simulink subsystem "StudentTemplate_NGCMAN017_M1"  (R2025a)
settings: Solver=VariableStepAuto  StartTime=0.0  StopTime=10.0  RelTol=1e-3
libraries: eeGeneralControl x3, simulink x2, slpidlib x1
settings Model: Creator=JesseJabezArendse  LastModifiedBy=Manelisi Ngcobo

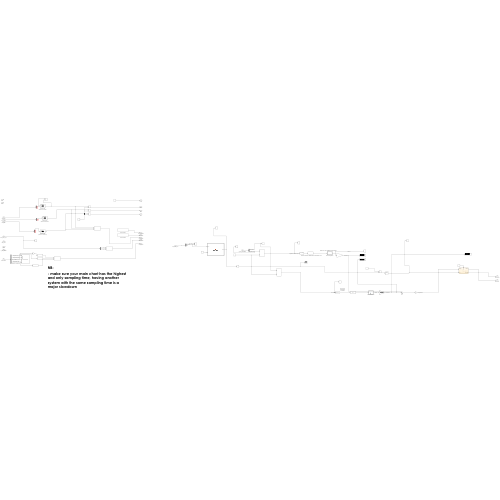
[thumbnail: Simulink's stored preview of the top-level diagram]
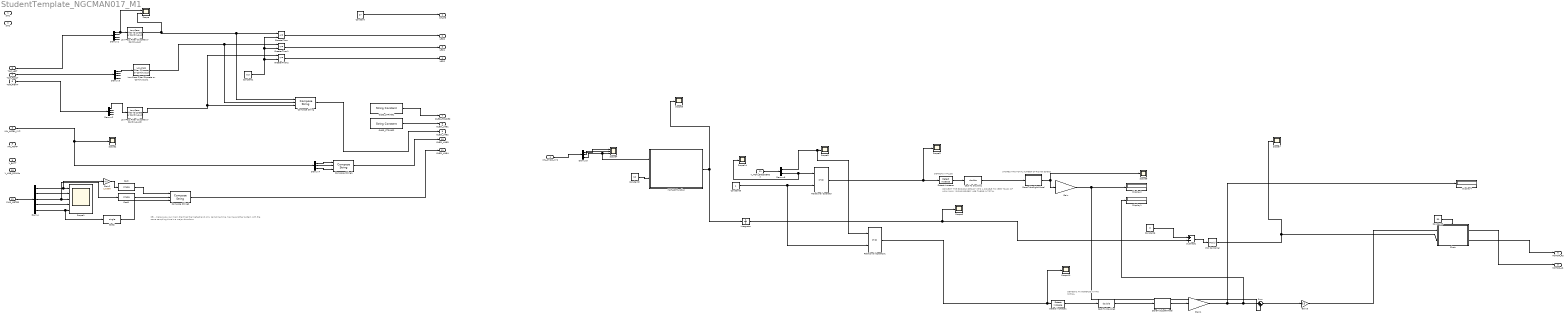
== system StudentTemplate_NGCMAN017_M1 ==
  note: NB:
      |
      | - make sure your main chart has the highest and only sampling time, having another system with the same sampling time is a major slowdown
  note: STORES THE TOTAL NUMBER OF RISING EDGES
  note: DETECTS AN INCREASE IN THE SIGNAL
  note: DETECTS A PULSE
  note: CONVERT THE BOOLEAN RESULT INTO A DOUBLE TO KEEP TRACK OF HOW MANY "RISING EDGES" ARE THERE IN TOTAL
  SW1 : Inport
  SW2 : Inport  Port=2
  IMU_ACCEL_XYZ : Inport  Port=3
  IMU_GYRO_XYZ : Inport  Port=4
  IMU_TEMP : Inport  Port=5
  TOF_LEFT : Inport  Port=6
  TOF_FRONT : Inport  Port=7
  TOF_RIGHT : Inport  Port=8
  V_BATT : Inport  Port=9
  V_LINE_DOWNs : Inport  Port=10
  V_MOT_ENCODERSs : Inport  Port=11
  PWR_METER : Inport  Port=12
  Cast : DataTypeConversion  OutDataTypeStr=single  SaturateOnIntegerOverflow=off  RndMeth=Floor
  Cast To Double1 : DataTypeConversion  OutDataTypeStr=double  SaturateOnIntegerOverflow=off  RndMeth=Floor
  Cast To Double2 : DataTypeConversion  OutDataTypeStr=double  SaturateOnIntegerOverflow=off  RndMeth=Floor
  Cast1 : DataTypeConversion  OutDataTypeStr=single  SaturateOnIntegerOverflow=off  RndMeth=Floor
  Cast2 : DataTypeConversion  OutDataTypeStr=single  SaturateOnIntegerOverflow=off  RndMeth=Floor
  Chart : Stateflow chart  TreatAsAtomicUnit=on
      settings: PortSchema="{\"entries\":[{\"content\":{\"sides\":[{\"content\":{\"connectorIds\":[\"In2\",\"In3\"]},\"type\":\"ConnectorPlacement.EquallySpacedRectSide\",\"uuid\":\"a71d10d4-7769-4bd5-a4c8-3911887a0d2d\"},{\"content\":{\"connectorIds\":[\"Out1\",\"Out2\"],\"side\":\"RIGHT\"},\"type\":\"ConnectorPlacement.EquallySpacedRectSide\",\"uuid\":\"f2808692-454e-4cab-a96d-7bb0cece0bc7\"},{\"content\":{\"connectorIds\":[\"In1\"],\"side\":\"TOP\"},\"type\":\"ConnectorPlacement.EquallySpacedRectSide\",\"uuid\":\"b188f5e3-29a6-4590-b94a-306fec8e8165\"}]},\"type\":\"ConnectorPlacement.EquallySpacedConnector\",\"uuid\":\"72d5cd91-91a4-4a68-a786-e95fb8ebc238\"}],\"packageUris\":[\"http://schema.mathworks.com/mf0/Connector/R2020b\"],\"version\":\"1.0\"}"
  Compose String : ComposeString  Format="\"L%1.2f F%1.2f R%1.2f\""
  Compose String1 : ComposeString  Format="\"X%2.1f  Y%2.1f  Z%2.1f\""
  Compose String2 : ComposeString  Format="\"%1.2fV  %3.0fmA  %2.0f%%\""
  Constant : Constant  Value=27
  Constant1 : Constant  Value=0.3  SampleTime=-1
  Constant2 : Constant  Value=10
  Constant3 : Constant  Value=50
  Constant5 : Constant
  Constant6 : Constant  Value=0
  Demux : Demux  Outputs=5
  Demux1 : Demux
  Demux2 : Demux
  Demux3 : Demux
  Demux4 : Demux  Outputs=3
  Demux5 : Demux  Outputs=3
  Demux6 : Demux  Outputs=2
  Detect Increase : simulink/Logic and Bit Operations/Detect Increase  vinit=0.0  OutDataTypeStr=boolean
  Detect Increase1 : simulink/Logic and Bit Operations/Detect Increase  vinit=0.0  OutDataTypeStr=boolean
  Display1 : Display
  Display2 : Display
  Display4 : Display
  Gain : Gain  Gain=0.25*pi*0.031
  Gain1 : Gain  Gain=0.25*pi*0.031
  Gain2 : Gain  Gain=1/1000
  Gain3 : Gain  Gain=0.5
  GreaterThan : RelationalOperator  Operator=<=  OutDataTypeStr=boolean  RndMeth=Simplest  InputSameDT=off
  GreaterThan1 : RelationalOperator  Operator=<=  OutDataTypeStr=boolean  RndMeth=Simplest  InputSameDT=off
  GreaterThan2 : RelationalOperator  Operator=<=  OutDataTypeStr=boolean  RndMeth=Simplest  InputSameDT=off
  Integrator : Integrator
  Low-Pass Filter (Discrete or Continuous) : eeGeneralControl/Low-Pass Filter (Discrete or Continuous)  K=1  T=0.1  B=inf  A=-inf  init_option=Inherited from block input  x0=0  Ts=-1
  Low-Pass Filter (Discrete or Continuous)1 : eeGeneralControl/Low-Pass Filter (Discrete or Continuous)  K=1  T=0.1  B=inf  A=-inf  init_option=Inherited from block input  x0=0  Ts=-1
  Low-Pass Filter (Discrete or Continuous)2 : eeGeneralControl/Low-Pass Filter (Discrete or Continuous)  K=1  T=0.1  B=inf  A=-inf  init_option=Inherited from block input  x0=0  Ts=-1
  MATLAB Function : MATLAB Function  TreatAsAtomicUnit=on
  OLED_STRING1 : StringConstant  String="\"UCT MICROMOUSE '25\""
  OLED_STRING2 : StringConstant  String="\"Simulink Data Demo\""
  PID Controller : slpidlib/PID Controller  Controller=PID  Form=Parallel  TimeDomain=Continuous-time  UseExternalTs=off  SampleTime=-1  IntegratorMethod=Forward Euler  FilterMethod=Forward Euler  ControllerParametersSource=internal  P=-0.30  I=0  UseKiTs=off  D=0  UseExternalDerivativeSource=off  N=100  UseFilter=on  TunerSelectOption=Transfer Function Based (PID Tuner App)  InitialConditionSource=internal  InitialConditionForIntegrator=0  InitialConditionForFilter=0  DifferentiatorICPrevScaledInput=0  ExternalReset=none  TrackingMode=off  Kt=1  LimitOutput=off  SatLimitsSource=internal  UpperSaturationLimit=inf  LowerSaturationLimit=-inf  LinearizeAsGain=on  AntiWindupMode=none  Kb=1  LimitIntegrator=off  UpperIntegratorSaturationLimit=inf  LowerIntegratorSaturationLimit=-inf  POutMin=[]  POutMax=[]  IOutMin=[]  IOutMax=[]  DOutMin=[]  DOutMax=[]  NOutMin=[]  NOutMax=[]  SumOutMin=[]  SumOutMax=[]  SaturationOutMin=[]  SaturationOutMax=[]  PParamMin=[]  PParamMax=[]  IParamMin=[]  IParamMax=[]  DParamMin=[]  DParamMax=[]  NParamMin=[]  NParamMax=[]  KbParamMin=[]  KbParamMax=[]  KtParamMin=[]  KtParamMax=[]  KbOutMin=[]  KbOutMax=[]  KtOutMin=[]  KtOutMax=[]  IntegratorOutMin=[]  IntegratorOutMax=[]  FilterOutMin=[]  FilterOutMax=[]  SumI1OutMin=[]  SumI1OutMax=[]  SumI2OutMin=[]  SumI2OutMax=[]  SumI3OutMin=[]  SumI3OutMax=[]  SumI4OutMin=[]  SumI4OutMax=[]  SumDOutMin=[]  SumDOutMax=[]  DifferentiatorOutMin=[]  DifferentiatorOutMax=[]  FilterDiffOutCoefMin=[]  FilterDiffOutCoefMax=[]  ReciprocalOutMin=[]  ReciprocalOutMax=[]  SumDenOutMin=[]  SumDenOutMax=[]  SumNumOutMin=[]  SumNumOutMax=[]  DivideOutMin=[]  DivideOutMax=[]  UdiffTsProdOutMin=[]  UdiffTsProdOutMax=[]  NTsProdOutMin=[]  NTsProdOutMax=[]  UintegralTsProdOutMin=[]  UintegralTsProdOutMax=[]  UngainTsProdOutMin=[]  UngainTsProdOutMax=[]  ClampingZeroOutDataTypeStr=Inherit: Inherit via back propagation  ClampingZeroOutMin=[]  ClampingZeroOutMax=[]  FilterDenConstantOutDataTypeStr=Inherit: Inherit via back propagation  FilterDenConstantOutMin=[]  FilterDenConstantOutMax=[]  PCopyOutDataTypeStr=Inherit: Inherit via back propagation  PCopyOutMin=[]  PCopyOutMax=[]  NCopyOutDataTypeStr=Inherit: Inherit via back propagation  NCopyOutMin=[]  NCopyOutMax=[]  IntegratorContinuousStateAttributes=''  IntegratorStateMustResolveToSignalObject=off  IntegratorRTWStateStorageClass=Auto  FilterContinuousStateAttributes=''  FilterStateMustResolveToSignalObject=off  FilterRTWStateStorageClass=Auto  ParallelPVariant=InternalParameters  IdealPVariant=Disabled  IVariant=InternalParameters  DVariant=InternalParameters  IntegratorVariant=Continuous  SatVariant=Disabled  AWVariant=Passthrough  PCopyVariant=Disabled  TRVariant=Disabled  FdbkBlocksVariant=Forward  IdealPFdbkVariant=Disabled  SatFdbkVariant=Disabled  DerivativeFilterVariant=ContFilter  NVariant=InternalParameters  NCopyVariant=Disabled  FilterICVariant=InternalICsFilter  IntegratorICVariant=InternalICs  ExternalResetVariant=Disabled  TRSumVariant=Passthrough  SumFdbkVariant=Disabled  SumVariant=Sum_PID  TsampFilterVariant=InternalTs  TsampNgainVariant=Passthrough  TsampIntegralVariant=Disabled_SignalSpec  ExternalSaturationOutDataTypeStr=Inherit: Same as second input  DerivativeSourceVariant=ErrorSignal  PreIntVariant=InternalPreInt
  Relational Operator : RelationalOperator  OutDataTypeStr=boolean  RndMeth=Simplest  InputSameDT=off
  Relational Operator1 : RelationalOperator  OutDataTypeStr=boolean  RndMeth=Simplest  InputSameDT=off
  Scope : Scope  NumInputPorts=2
      settings: ActiveDisplayYMinimum=0.22759  ActiveDisplayYMaximum=0.52326
  Scope1 : Scope  NumInputPorts=5
      settings: ActiveDisplayYMinimum=-437.5  ActiveDisplayYMaximum=3937.5  DataLoggingVariableName=ScopeData2
  Scope{2..3,5..10,14} (9 alike) : Scope
      Scope10 settings: ActiveDisplayYMinimum=-0.12499999999999997  ActiveDisplayYMaximum=1.125  DataLoggingVariableName=ScopeData11
      Scope14 settings: ActiveDisplayYMinimum=0.33824470727261841  ActiveDisplayYMaximum=0.45617059888922451  DataLoggingVariableName=ScopeData16
      Scope3 settings: ActiveDisplayYMinimum=-0.12499999999999997  ActiveDisplayYMaximum=1.125  DataLoggingVariableName=ScopeData4
      Scope5 settings: ActiveDisplayYMinimum=-71.808765356003278  ActiveDisplayYMaximum=72.321645335275264  DataLoggingVariableName=ScopeData5
      Scope6 settings: ActiveDisplayYMinimum=-0.034238451185607394  ActiveDisplayYMaximum=0.30814606067046663  DataLoggingVariableName=ScopeData6
      Scope7 settings: ActiveDisplayYMinimum=-1  ActiveDisplayYMaximum=1  DataLoggingVariableName=ScopeData7
      Scope8 settings: ActiveDisplayYMinimum=-0.74999999999999978  ActiveDisplayYMaximum=6.75  DataLoggingVariableName=ScopeData12
      Scope9 settings: ActiveDisplayYMinimum=-0.12499999999999997  ActiveDisplayYMaximum=1.125  DataLoggingVariableName=ScopeData8
  Scope4 : Scope  NumInputPorts=3
      settings: ActiveDisplayYMinimum=-0.29194188682177158  ActiveDisplayYMaximum=0.282998724531242  DataLoggingVariableName=ScopeData3
  StoreTicksLeftWheel : MATLAB Function  TreatAsAtomicUnit=on
  StoreTicksRightWheel : MATLAB Function  TreatAsAtomicUnit=on
  Subtract1 : Sum  Inputs=+-
  Sum : Sum  Inputs=|++
  STATE : Outport
  LED0 : Outport  Port=2
  LED1 : Outport  Port=3
  LED2 : Outport  Port=4
  MOTOR_LS : Outport  Port=5
  MOTOR_RS : Outport  Port=6
  OLED_HEADER : Outport  Port=7
  OLED_LINE1 : Outport  Port=8
  OLED_LINE2 : Outport  Port=9
  OLED_LINE3 : Outport  Port=10
  OLED_LINE4 : Outport  Port=11
  wires:
  TOF_FRONT/1 -> Demux3/1
  OLED_STRING2/1 -> OLED_LINE1/1
  Demux2/1 -> Low-Pass Filter (Discrete or Continuous)2/1
  Demux2/3 -> ?
  Demux2/2 -> ?
  Demux2/4 -> ?
  Compose String1/1 -> OLED_LINE3/1
  Low-Pass Filter (Discrete or Continuous)1/1 -> Compose String/2, GreaterThan1/1
  GreaterThan1/1 -> LED1/1
  Demux3/3 -> ?
  TOF_RIGHT/1 -> Demux2/1
  Demux3/4 -> ?
  Demux3/2 -> ?
  Demux1/2 -> ?
  Demux3/1 -> Low-Pass Filter (Discrete or Continuous)1/1
  OLED_STRING1/1 -> OLED_HEADER/1
  Demux1/1 -> Scope/1, Low-Pass Filter (Discrete or Continuous)/1
  Compose String/1 -> OLED_LINE2/1
  Constant1/1 -> GreaterThan2/2, GreaterThan1/2, GreaterThan/2
  Demux1/4 -> ?
  GreaterThan2/1 -> LED2/1
  TOF_LEFT/1 -> Demux1/1
  GreaterThan/1 -> LED0/1
  Demux1/3 -> ?
  PWR_METER/1 -> Demux/1
  Demux/1 -> Scope1/1, Gain2/1  "PWR_VBATT [mV]"
  Demux/2 -> Scope1/2  "PWR_VSHUNT [mV]"
  Demux/3 -> Scope1/3, Cast1/1  "PWR_CURRENT [mA]"
  Demux/4 -> Scope1/4  "PWR_POWER [mW]"
  Demux/5 -> Scope1/5, Cast2/1  "PWR_BATT_PERCENT [%]"
  IMU_ACCEL_XYZ/1 -> Demux4/1, Scope2/1
  Demux4/1 -> Compose String1/1
  Demux4/2 -> Compose String1/2
  Demux4/3 -> Compose String1/3
  Compose String2/1 -> OLED_LINE4/1
  Gain2/1 -> Cast/1
  Cast/1 -> Compose String2/1
  Cast1/1 -> Compose String2/2
  Cast2/1 -> Compose String2/3
  Low-Pass Filter (Discrete or Continuous)2/1 -> Compose String/3, GreaterThan2/1
  Low-Pass Filter (Discrete or Continuous)/1 -> Scope/2, Compose String/1, GreaterThan/1
  Constant/1 -> STATE/1
  Gain1/1 -> Display4/1, Display1/1, Sum/1  "TotalDistance"
  Detect Increase/1 -> Cast To Double1/1
  StoreTicksLeftWheel/1(y) -> Gain1/1  "TotalTicks"
  Cast To Double2/1 -> StoreTicksLeftWheel/1(u)
  Demux6/2 -> Scope14/1, Relational Operator/1  "RightWheelOut"
  Subtract1/1 -> PID Controller/1
  Relational Operator/1 -> Detect Increase/1, Scope3/1  "RightMotorEncoderOutToSquare"
  Sum/1 -> Gain3/1
  Gain/1 -> Sum/2, Display2/1  "TotalDistance"
  StoreTicksRightWheel/1(y) -> Scope8/1, Gain/1  "TotalTicks"
  Constant5/1 -> Relational Operator1/2, Relational Operator/2
  Gain3/1 -> Chart/2(AveDist)  "AverageDistance"
  PID Controller/1 -> Scope7/1, Chart/3(error)
  Constant6/1 -> Subtract1/1
  Detect Increase1/1 -> Cast To Double2/1
  Relational Operator1/1 -> Detect Increase1/1, Scope10/1  "MotorEncoderOut"
  Cast To Double1/1 -> StoreTicksRightWheel/1(u)
  Demux6/1 -> Relational Operator1/1, Scope9/1  "LeftWheelOut"
  V_MOT_ENCODERSs/1 -> Demux6/1
  IMU_GYRO_XYZ/1 -> Demux5/1
  Demux5/1 -> Scope4/1  "X"
  Demux5/2 -> Scope4/2  "Y"
  Demux5/3 -> Scope4/3, MATLAB Function/1(gyroZ)  "Z"
  Constant2/1 -> MATLAB Function/2(dt)
  Integrator/1 -> Scope6/1, Subtract1/2
  MATLAB Function/1(theta) -> Scope5/1, Integrator/1
  Chart/1(MotorLS) -> MOTOR_LS/1
  Chart/2(MotorRS) -> MOTOR_RS/1
  Constant3/1 -> Chart/1(Speed)

== matlab function StudentTemplate_NGCMAN017_M1/StoreTicksRightWheel ==
  settings: updateMethod=DISCRETE
  data: u input; y output
function y = fcn(u)
persistent prevHigh count

if isempty(prevHigh)
    prevHigh = false;  % previous high state
    count = 0;         % initialize counter
end

% ensure scalar for logical operations
u_scalar = u(1);

threshold = 0.5;          % define threshold
isHigh = u_scalar > threshold;   % detect high state

% detect rising edge
if isHigh && ~prevHigh
    count = count + 1;
end

y = count;         % output current count
prevHigh = isHigh; % update previous state
end

== stateflow chart StudentTemplate_NGCMAN017_M1/Chart ==
  state MoveForward
    during:
    MotorRS = Speed-error;
    MotorLS = Speed+error;
  state Stop
    entry:
    MotorRS = 0;
    MotorLS = 0;
  (default) -> MoveForward
  MoveForward -> Stop : [AveDist>=2]
  data: Speed input; MotorLS output; MotorRS output; AveDist input; error input

== matlab function StudentTemplate_NGCMAN017_M1/MATLAB Function ==
  settings: updateMethod=DISCRETE
  data: gyroZ input; theta output; dt input
function theta = gyroYawCorrected(gyroZ, dt)
%#codegen
% Computes yaw angle (theta) from gyro Z with automatic bias removal.
% Uses first 2 seconds for calibration, then integrates corrected signal.
%
% Inputs:
%   gyroZ - gyro Z axis (rad/s) (scalar)
%   dt    - sample time (s)
% Output:
%   theta - yaw angle (rad), corrected

% Force inputs to double
gyroZ = double(gyroZ);
dt    = double(dt);

% Persistent variables
persistent biasEst count sumSamples calibrated theta_prev
if isempty(biasEst)
    biasEst    = 0;
    count      = 0;
    sumSamples = 0;
    calibrated = false;
    theta_prev = 0;
end

% Update counters
count = count + 1;
sumSamples = sumSamples + gyroZ;

% --- Calibration phase (first 2 seconds) ---
if ~calibrated
    if count*dt >= 1
        biasEst = sumSamples / count; % compute gyro bias
        calibrated = true;
    end
    theta = 0; % keep theta = 0 until calibration done
    return
end

% --- Bias correction ---
gyroCorr = gyroZ - biasEst;

% --- Integrate gyro to get yaw ---
theta = theta_prev + gyroCorr * dt;

% Save state
theta_prev = theta;
end

== matlab function StudentTemplate_NGCMAN017_M1/StoreTicksLeftWheel ==
  settings: updateMethod=DISCRETE
  data: u input; y output
function y = fcn(u)
persistent prevHigh count

if isempty(prevHigh)
    prevHigh = false;  % previous high state
    count = 0;         % initialize counter
end

% ensure scalar for logical operations
u_scalar = u(1);

threshold = 0.5;          % define threshold
isHigh = u_scalar > threshold;   % detect high state

% detect rising edge
if isHigh && ~prevHigh
    count = count + 1;
end

y = count;         % output current count
prevHigh = isHigh; % update previous state
end
